simulink model "triping"  (R2025b)
settings: Solver=VariableStepAuto  StartTime=0.0  StopTime=10.0  RelTol=1e-3
settings Model: Creator=Dell  LastModifiedBy=Dell

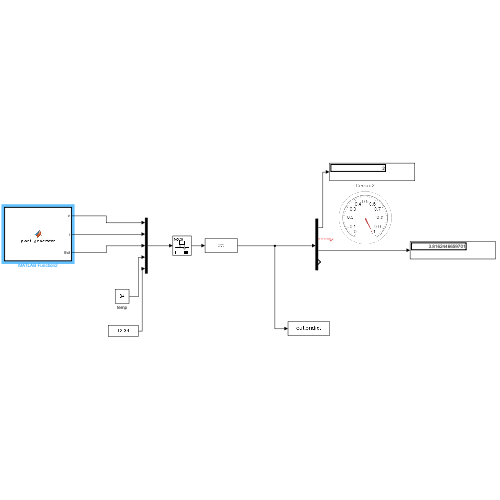
[thumbnail: Simulink's stored preview of the top-level diagram]
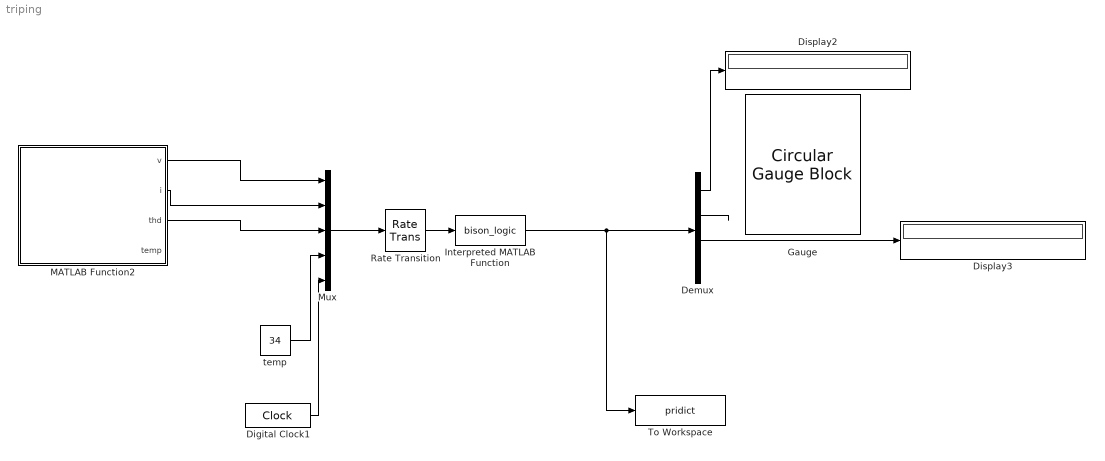
== system triping ==
  Demux : Demux
  Digital Clock1 : DigitalClock  SampleTime=0.05
  Display2 : Display
      settings: Format=decimal (Stored Integer)
  Display3 : Display
      settings: Format=decimal (Stored Integer)
  Gauge : CircularGaugeBlock  ScaleMax=1  TickInterval=0.1  FontColor=[0.0, 0.0, 0.0]
  Interpreted MATLAB Function : MATLABFcn  MATLABFcn=bison_logic
  MATLAB Function2 : MATLAB Function  TreatAsAtomicUnit=on
  Mux : Mux  Inputs=5
  Rate Transition : RateTransition  OutPortSampleTime=0.05
  To Workspace : ToWorkspace  VariableName=pridict  SaveFormat=Timeseries  SampleTime=-1
  temp : Constant  Value=34
  wires:
  Demux/1 -> Display2/1
  Demux/3 -> Display3/1
  Digital Clock1/1 -> Mux/5
  Interpreted MATLAB Function/1 -> To Workspace/1, Demux/1
  MATLAB Function2/1(v) -> Mux/1
  MATLAB Function2/2(i) -> Mux/2
  MATLAB Function2/3(thd) -> Mux/3
  temp/1 -> Mux/4
  Mux/1 -> Rate Transition/1
  Rate Transition/1 -> Interpreted MATLAB Function/1
  Demux/2 -> ?

== matlab function triping/MATLAB Function2 ==
  data: v output; i output; thd output; temp output
function [v, i, thd, temp] = plant_generator()
    persistent count;
    if isempty(count), count = 1; end
    
    N_total = 5000;
    % Natural fluctuations based on your CSV characteristics
    v_n = (rand - 0.5) * 0.4; 
    i_n = (rand - 0.5) * 0.15;
    t_n = (rand - 0.5) * 0.1;

    % --- DYNAMIC PATTERN GENERATION ---
    % Pattern 1 (Low) and Pattern 2 (Medium) alternate to simulate 
    % varying loads on an EV charging station.
    if mod(count, 150) < 75
        % LOW SPIKE PATTERN (Stable Operation)
        v = 24.2 + v_n; 
        i = 1.8 + i_n; 
        thd = 0.25 + (rand*0.02); 
        temp = 35.0 + (count/1000);
    else
        % MEDIUM SPIKE PATTERN (Pre-Fault Stress)
        % This is the pattern the AI will use to predict a High Spike
        v = 28.5 + v_n; 
        i = 7.5 + i_n; 
        thd = 0.35 + (rand*0.05); 
        temp = 45.0 + (count/500);
    end
    
    if count < N_total, count = count + 1; end
end
